simulink model "two_spring_mass_damper_system_simulink"  (R2019b)
settings: Solver=VariableStepAuto  StartTime=0.0  StopTime=10  RelTol=1e-3
values from neighbouring files (symbols this model uses):
  c1 = 100    [two_spring_mass_damper_system.m]
  c2 = 1000    [two_spring_mass_damper_system.m]
  k1 = 1e4    (= 10000)    [two_spring_mass_damper_system.m]
  k2 = 1e5    (= 100000)    [two_spring_mass_damper_system.m]
  m1 = 10    [two_spring_mass_damper_system.m]
  m2 = 100    [two_spring_mass_damper_system.m]
settings Model: Creator=sahil  LastModifiedBy=sahil

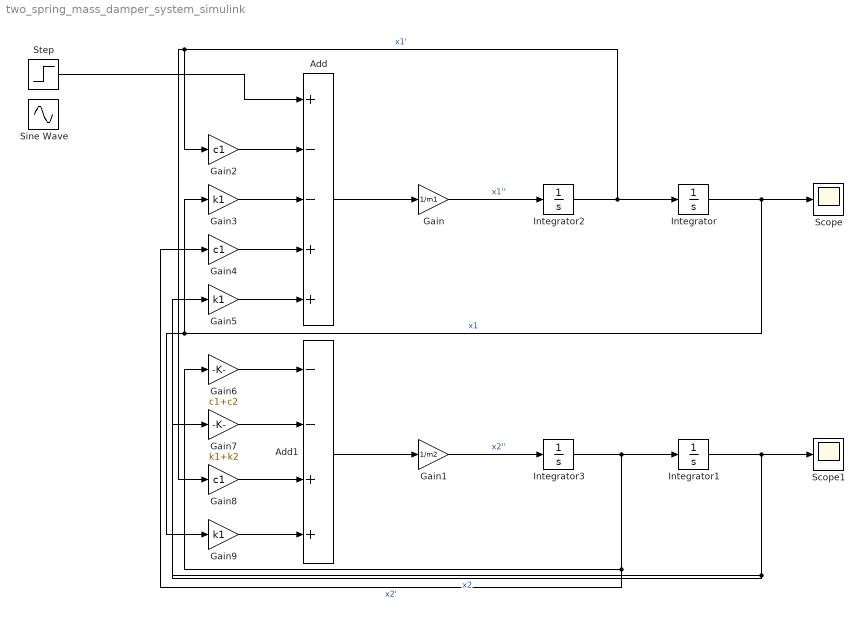
== system two_spring_mass_damper_system_simulink ==
  Add : Sum  Inputs=+--++
  Add1 : Sum  Inputs=--++
  Gain : Gain  Gain=1/m1
  Gain1 : Gain  Gain=1/m2
  Gain2 : Gain  Gain=c1
  Gain3 : Gain  Gain=k1
  Gain4 : Gain  Gain=c1
  Gain5 : Gain  Gain=k1
  Gain6 : Gain  Gain=c1+c2
  Gain7 : Gain  Gain=k1+k2
  Gain8 : Gain  Gain=c1
  Gain9 : Gain  Gain=k1
  Integrator{,1..3} (4 alike) : Integrator
  Scope : Scope
  Scope1 : Scope
  Sine Wave : Sin  Amplitude=3  Frequency=10  SampleTime=0
  Step : Step  Time=0  After=5  SampleTime=0
  wires:
  Integrator/1 -> Gain9/1, Gain3/1, Scope/1  "x1"
  Integrator1/1 -> Gain7/1, Gain5/1, Scope1/1  "x2"
  Integrator3/1 -> Gain6/1, Gain4/1, Integrator1/1  "x2'"
  Integrator2/1 -> Gain8/1, Gain2/1, Integrator/1  "x1'"
  Gain/1 -> Integrator2/1  "x1''"
  Gain1/1 -> Integrator3/1  "x2''"
  Add/1 -> Gain/1
  Gain2/1 -> Add/2
  Gain3/1 -> Add/3
  Gain6/1 -> Add1/1
  Gain7/1 -> Add1/2
  Gain8/1 -> Add1/3
  Gain9/1 -> Add1/4
  Add1/1 -> Gain1/1
  Gain5/1 -> Add/5
  Gain4/1 -> Add/4
  Step/1 -> Add/1
